simulink model "simulaciontorque"  (R2020b)
settings: Solver=VariableStepAuto  StartTime=0.0  StopTime=1.3  RelTol=1e-3
values from neighbouring files (symbols this model uses):
  beq = bm+(blnom/(r^2))    (= 1.5e-05)    [valores.m]
  Cts = 0.818    [Valores_de_Parametros.m]    (also in valores.m)
  Jeq = (Jm+Jl/r^2)    (= 5.65099476805e-06)    [Valores_de_Parametros.m]    (also in valores.m)
  lambda_m = 0.01546    [Valores_de_Parametros.m]    (also in valores.m)
  Ld = 6.6    [Valores_de_Parametros.m]    (also in valores.m = 0.0066)
  Lls = 0.8    [Valores_de_Parametros.m]    (also in valores.m = 0.0008)
  Lq = 5.8    [Valores_de_Parametros.m]    (also in valores.m = 0.0058)
  Pp = 3    [Valores_de_Parametros.m]    (also in valores.m)
  r = 314.3008    [Valores_de_Parametros.m]    (also in valores.m)
  R0 = Lls*pi    (= 4)    [valores.m]
  Rd = Ld*pi    (= 33)    [valores.m]
  Rq = Lq*pi    (= 29)    [valores.m]
  Rs = 1.02    [Valores_de_Parametros.m]    (also in valores.m)
  Rts_amb = 146.7    [Valores_de_Parametros.m]    (also in valores.m)
undefined symbols (not defined in the file or in its folder): sigbuilder_block
settings Model: Creator=Matias  LastModifiedBy=Matias

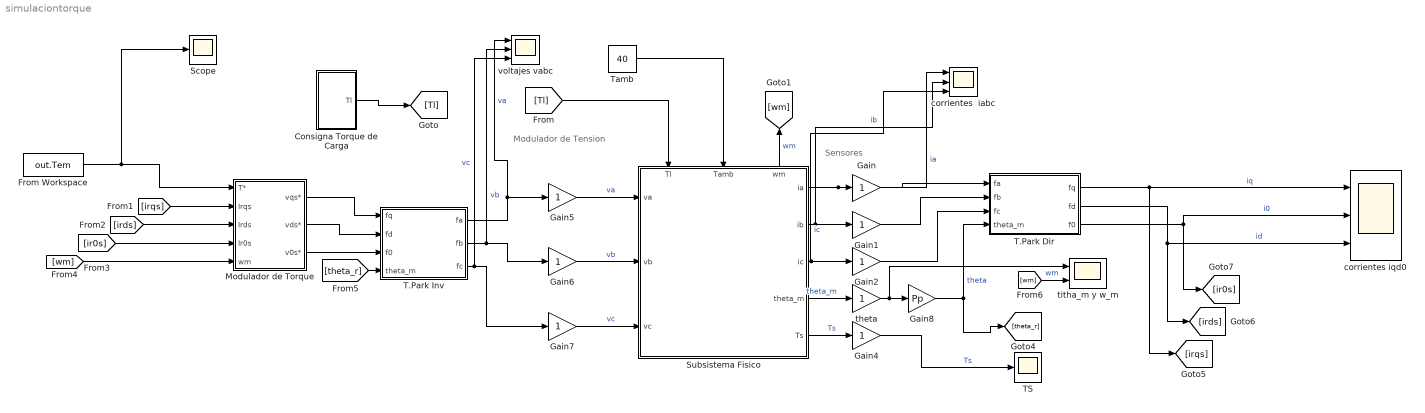
== system simulaciontorque ==
  note: Modulador de Tension
  note: Sensores
  Consigna Torque de Carga : Subsystem
  From Workspace : FromWorkspace  VariableName=out.Tem
  Gain{,1..2,4..7} (7 alike) : Gain
  Gain8 : Gain  Gain=Pp
  Modulador de Torque : Subsystem
  Scope : Scope
  Subsistema Fisico : Subsystem
      settings: PortSchema="{\"entries\":[{\"content\":{\"sides\":[{\"content\":{\"connectorIds\":[\"In1\",\"In2\",\"In3\"]},\"type\":\"ConnectorPlacement.EquallySpacedRectSide\",\"uuid\":\"428e53fe-c6d6-4999-95eb-db171c1d7752\"},{\"content\":{\"connectorIds\":[\"Out1\",\"Out2\",\"Out3\",\"Out4\",\"Out5\"],\"side\":\"RIGHT\"},\"type\":\"ConnectorPlacement.EquallySpacedRectSide\",\"uuid\":\"d3984cce-d898-4b9d-ab92-7967eebad5db\"},{\"content\":{\"connectorIds\":[\"In4\",\"In5\",\"Out6\"],\"side\":\"TOP\"},\"type\":\"ConnectorPlacement.EquallySpacedRectSide\",\"uuid\":\"4e08f4f3-ce82-4568-8c70-e26e1ed2ccd9\"},{\"content\":{\"connectorIds\":[],\"side\":\"BOTTOM\"},\"type\":\"ConnectorPlacement.EquallySpacedRectSide\",\"uuid\":\"f5359b7b-31c8-439d-9b4b-495d60398ac6\"},{\"content\":{\"connectorIds\":[],\"side\":\"HIDDEN\"},\"type\":\"ConnectorPlacement.EquallySpacedRectSide\",\"uuid\":\"fe5ef39c-0012-48bd-8627-0cf1abf153f6\"}]},\"type\":\"ConnectorPlacement.EquallySpacedConnector\",\"uuid\":\"3b2746a1-6d8c-49ea-8ba7-7e2e359e7a22\"}],\"packageUris\":[\"http://schema.mathworks.com/mf0/Connector/R2020b\"],\"version\":\"1.0\"}"
  T.Park Dir : MATLAB Function  TreatAsAtomicUnit=on
  T.Park Inv : MATLAB Function  TreatAsAtomicUnit=on
  TS : Scope
  Tamb : Constant  Value=40
  corrientes  iabc : Scope  NumInputPorts=3
  corrientes iqd0 : Scope  NumInputPorts=3
  theta : Gain
  titha_m y w_m : Scope  NumInputPorts=2
  voltajes vabc : Scope  NumInputPorts=3
  wires:
  Tamb/1 -> Subsistema Fisico/5(Tamb)
  [theta_r] -> T.Park Inv/4(theta_m)
  Modulador de Torque/1(vqs*) -> T.Park Inv/1(fq)
  [irds] -> Modulador de Torque/3(Irds)
  [ir0s] -> Modulador de Torque/4(Ir0s)
  Gain/1 -> T.Park Dir/1(fa)
  Modulador de Torque/2(vds*) -> T.Park Inv/2(fd)
  T.Park Inv/1(fa) -> voltajes vabc/1, Gain5/1  "va"
  T.Park Inv/2(fb) -> voltajes vabc/2, Gain6/1  "vb"
  [Tl] -> Subsistema Fisico/4(Tl)
  Gain4/1 -> TS/1  "Ts"
  theta/1 -> titha_m y w_m/1, Gain8/1
  T.Park Dir/2(fd) -> [irds], corrientes iqd0/3  "id"
  T.Park Dir/1(fq) -> [irqs], corrientes iqd0/1  "iq"
  Subsistema Fisico/1(ia) -> corrientes  iabc/1, Gain/1  "ia"
  Subsistema Fisico/2(ib) -> corrientes  iabc/2, Gain1/1  "ib"
  Gain5/1 -> Subsistema Fisico/1(va)  "va"
  Gain7/1 -> Subsistema Fisico/3(vc)  "vc"
  Subsistema Fisico/6(wm) -> [wm]  "wm"
  Gain6/1 -> Subsistema Fisico/2(vb)  "vb"
  T.Park Dir/3(f0) -> [ir0s], corrientes iqd0/2  "i0"
  T.Park Inv/3(fc) -> voltajes vabc/3, Gain7/1  "vc"
  Gain8/1 -> T.Park Dir/4(theta_m), [theta_r]  "theta"
  [wm] -> titha_m y w_m/2  "wm"
  Gain2/1 -> T.Park Dir/3(fc)
  Subsistema Fisico/3(ic) -> corrientes  iabc/3, Gain2/1  "ic"
  Subsistema Fisico/4(theta_m) -> theta/1  "theta_m"
  Subsistema Fisico/5(Ts) -> Gain4/1  "Ts"
  Modulador de Torque/3(v0s*) -> T.Park Inv/3(f0)
  [wm] -> Modulador de Torque/5(wm)
  Gain1/1 -> T.Park Dir/2(fb)
  [irqs] -> Modulador de Torque/2(Irqs)
  From Workspace/1 -> Scope/1, Modulador de Torque/1(T*)
  Consigna Torque de Carga/1(Tl) -> [Tl]

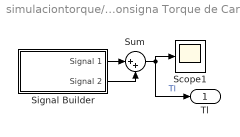
== system simulaciontorque/Consigna Torque de Carga ==
  Scope1 : Scope
  Signal Builder : Subsystem  Tag=STV Subsys  LoadFcn=sigbuilder_block('load');  StartFcn=sigbuilder_block('start');  StopFcn=sigbuilder_block('stop');  ClipboardFcn=sigbuilder_block('clipboard');  mask(Sigbuilder block){tuvar=[0:10]}
      mask help: Simulink:masks:SigbuilderBlock_MD
      mask init:
      | if ~strcmp(get_param(bdroot(gcbh),'SimulationStatus'),'stopped') tuvar = sigbuilder_block('maskInit'); end
      settings: CopyFcn=sigbuilder_block('copy');  DeleteFcn=sigbuilder_block('delete');  ModelCloseFcn=sigbuilder_block('modelClose');  PreSaveFcn=sigbuilder_block('preSave');  PauseFcn=sigbuilder_block('pause');  ContinueFcn=sigbuilder_block('continue');  NameChangeFcn=sigbuilder_block('namechange');  OpenFcn=sigbuilder_block('open',[388.2 64.2 550.8 400.2 ]);  CloseFcn=sigbuilder_block('close');
      mask Display: plot(0, 0, 100, 100,[2, 2, 32, 32, 2], [68, 8, 8, 68, 68],[32, 2], [38, 38], [32, 19, 2],[53, 60, 44], [32, 17, 17, 2],[16, 16, 31, 31]);txt = getActiveGroup(gcbh);text(2, 100, txt,'verticalAlignment', 'top');
  Sum : Sum  Inputs=|++
  Tl : Outport
  wires:
  Signal Builder/2(Signal 2) -> Sum/2
  Sum/1 -> Tl/1, Scope1/1  "Tl"
  Signal Builder/1(Signal 1) -> Sum/1

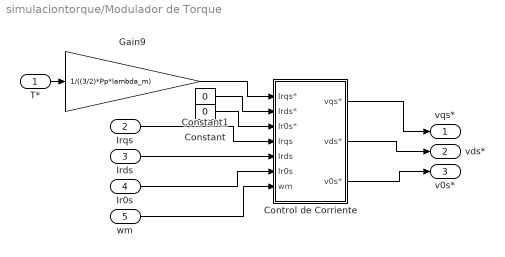
== system simulaciontorque/Modulador de Torque ==
  T* : Inport
  Irqs : Inport  Port=2
  Irds : Inport  Port=3
  Ir0s : Inport  Port=4
  wm : Inport  Port=5
  Constant : Constant  Value=0
  Constant1 : Constant  Value=0
  Control de Corriente : Subsystem
  Gain9 : Gain  Gain=1/((3/2)*Pp*lambda_m)
  vqs* : Outport
  vds* : Outport  Port=2
  v0s* : Outport  Port=3
  wires:
  Control de Corriente/2(vds*) -> vds*/1
  Irds/1 -> Control de Corriente/5(Irds)
  Gain9/1 -> Control de Corriente/1(Irqs*)
  Ir0s/1 -> Control de Corriente/6(Ir0s)
  Constant/1 -> Control de Corriente/3(Ir0s*)
  Control de Corriente/3(v0s*) -> v0s*/1
  Constant1/1 -> Control de Corriente/2(Irds*)
  Control de Corriente/1(vqs*) -> vqs*/1
  wm/1 -> Control de Corriente/7(wm)
  Irqs/1 -> Control de Corriente/4(Irqs)
  T*/1 -> Gain9/1

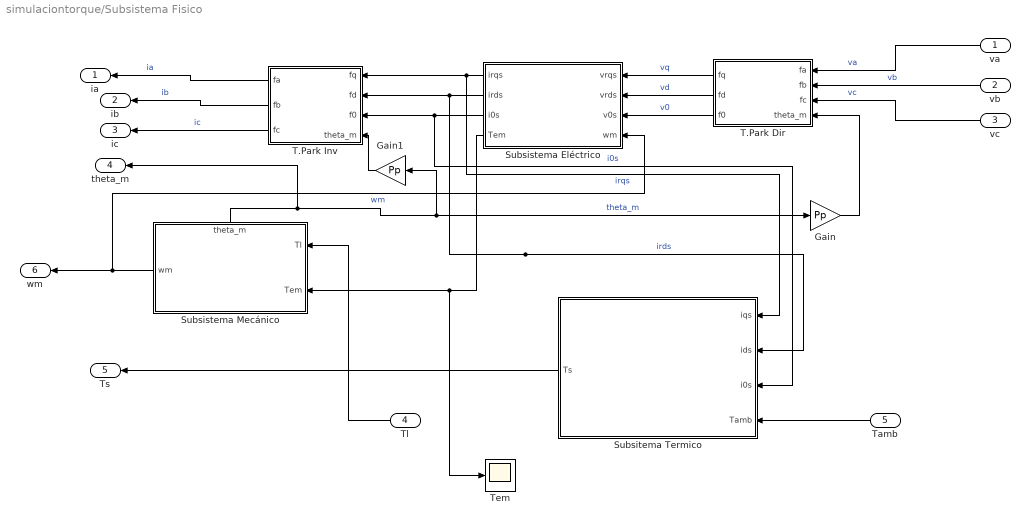
== system simulaciontorque/Subsistema Fisico ==
  va : Inport
  vb : Inport  Port=2
  vc : Inport  Port=3
  Tl : Inport  Port=4
  Tamb : Inport  Port=5
  Gain : Gain  Gain=Pp
  Gain1 : Gain  Gain=Pp
  Subsistema Eléctrico : Subsystem
  Subsistema Mecánico : Subsystem
      settings: PortSchema="{\"entries\":[{\"content\":{\"sides\":[{\"content\":{\"connectorIds\":[\"In1\",\"In2\"]},\"type\":\"ConnectorPlacement.EquallySpacedRectSide\",\"uuid\":\"ee0e19e9-1195-452b-ab3d-8be3dd040414\"},{\"content\":{\"connectorIds\":[\"Out1\"],\"side\":\"RIGHT\"},\"type\":\"ConnectorPlacement.EquallySpacedRectSide\",\"uuid\":\"524e54e6-4967-4b42-ae12-58774e9397a0\"},{\"content\":{\"connectorIds\":[\"Out2\"],\"side\":\"TOP\"},\"type\":\"ConnectorPlacement.EquallySpacedRectSide\",\"uuid\":\"fab71378-68cb-4446-b02c-df48705d1789\"},{\"content\":{\"connectorIds\":[],\"side\":\"HIDDEN\"},\"type\":\"ConnectorPlacement.EquallySpacedRectSide\",\"uuid\":\"eea92cb8-3517-43ef-96fe-10b46f054d59\"}]},\"type\":\"ConnectorPlacement.EquallySpacedConnector\",\"uuid\":\"156d3ac5-e5c7-4248-8590-4f82c7370a76\"}],\"packageUris\":[\"http://schema.mathworks.com/mf0/Connector/R2020b\"],\"version\":\"1.0\"}"
  Subsitema Termico : Subsystem
  T.Park Dir : MATLAB Function  TreatAsAtomicUnit=on
  T.Park Inv : MATLAB Function  TreatAsAtomicUnit=on
  Tem : Scope
  ia : Outport
  ib : Outport  Port=2
  ic : Outport  Port=3
  theta_m : Outport  Port=4
  Ts : Outport  Port=5
  wm : Outport  Port=6
  wires:
  Subsitema Termico/1(Ts) -> Ts/1
  Tl/1 -> Subsistema Mecánico/1(Tl)
  T.Park Inv/3(fc) -> ic/1  "ic"
  vb/1 -> T.Park Dir/2(fb)  "vb"
  Tamb/1 -> Subsitema Termico/4(Tamb)
  T.Park Inv/1(fa) -> ia/1  "ia"
  Subsistema Mecánico/1(wm) -> Subsistema Eléctrico/4(wm), wm/1  "wm"
  T.Park Dir/1(fq) -> Subsistema Eléctrico/1(vrqs)  "vq"
  Subsistema Eléctrico/3(i0s) -> Subsitema Termico/3(i0s), T.Park Inv/3(f0)  "i0s"
  Subsistema Eléctrico/1(irqs) -> Subsitema Termico/1(iqs), T.Park Inv/1(fq)  "irqs"
  Subsistema Eléctrico/2(irds) -> Subsitema Termico/2(ids), T.Park Inv/2(fd)  "irds"
  T.Park Dir/3(f0) -> Subsistema Eléctrico/3(v0s)  "v0"
  T.Park Dir/2(fd) -> Subsistema Eléctrico/2(vrds)  "vd"
  vc/1 -> T.Park Dir/3(fc)  "vc"
  T.Park Inv/2(fb) -> ib/1  "ib"
  Subsistema Mecánico/2(theta_m) -> theta_m/1, Gain1/1, Gain/1  "theta_m"
  va/1 -> T.Park Dir/1(fa)  "va"
  Subsistema Eléctrico/4(Tem) -> Tem/1, Subsistema Mecánico/2(Tem)
  Gain/1 -> T.Park Dir/4(theta_m)
  Gain1/1 -> T.Park Inv/4(theta_m)

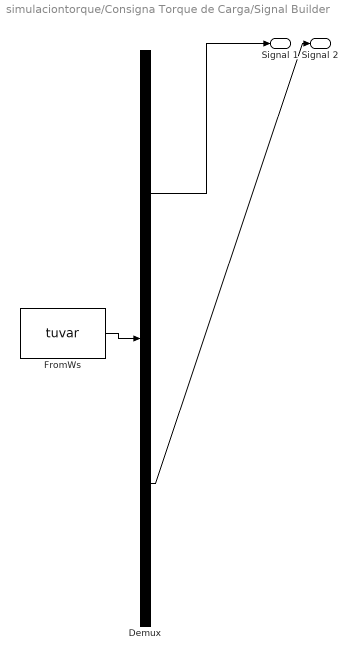
== system simulaciontorque/Consigna Torque de Carga/Signal Builder ==
  Demux : Demux  Tag=STV Demux  Outputs=2
      settings: DisplayOption=none
  FromWs : FromWorkspace  Tag=STV FromWs  VariableName=tuvar
      SigBuilderData=|
      | common.afterFinalStr = 'Extrapolate'
      | common.sampleTime = 0
      | dataSet.timeRange = [0 10]
      | dataSet.name = 'Group 1'
      | sbobj.Groups.Name = 'Group 1'
      | sbobj.Groups.Signals(1).Name = 'Signal 1'
      | sbobj.Groups.Signals(1).XData = [0 0.3 0.3 0.5 0.5 0.9 10]
      | sbobj.Groups.Signals(1).YData = [0 0 6.28 6.28 0 0 0]
      | sbobj.Groups.Signals(2).Name = 'Signal 2'
      | sbobj.Groups.Signals(2).XData = [0 0.5 0.5 0.9 0.9 10]
      | sbobj.Groups.Signals(2).YData = [0 0 -6.28 -6.28 0 0]
  Signal 1 : Outport  Tag=STV Outport
  Signal 2 : Outport  Tag=STV Outport  Port=2
  wires:
  Demux/1 -> Signal 1/1
  FromWs/1 -> Demux/1
  Demux/2 -> Signal 2/1

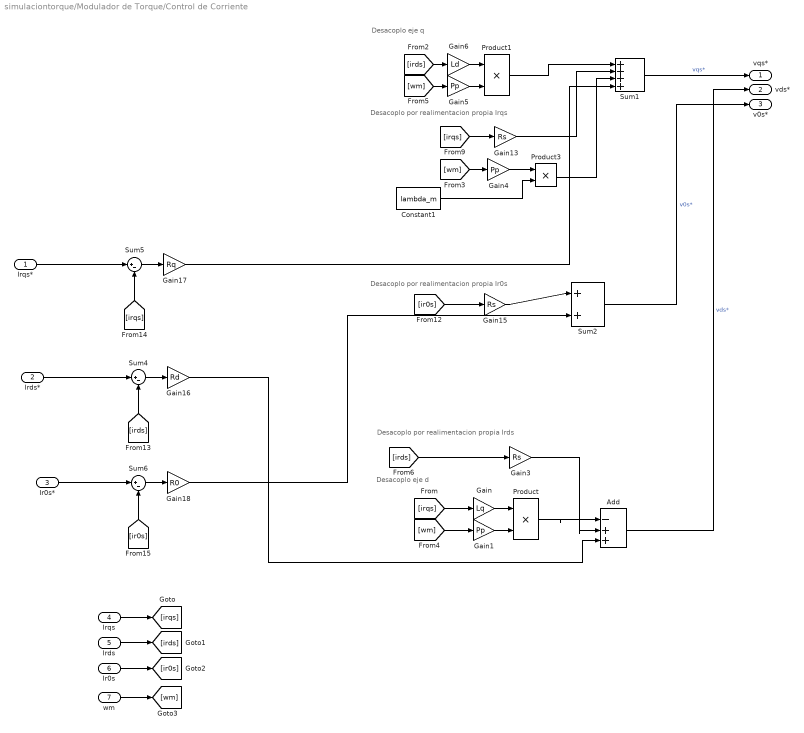
== system simulaciontorque/Modulador de Torque/Control de Corriente ==
  note: Desacoplo por realimentacion propia Ir0s
  note: Desacoplo por realimentacion propia Irqs
  note: Desacoplo por realimentacion propia Irds
  note: Desacoplo eje d
  note: Desacoplo eje q
  Irqs* : Inport
  Irds* : Inport  Port=2
  Ir0s* : Inport  Port=3
  Irqs : Inport  Port=4
  Irds : Inport  Port=5
  Ir0s : Inport  Port=6
  wm : Inport  Port=7
  Add : Sum  Inputs=|-++
  Constant1 : Constant  Value=lambda_m
  Gain : Gain  Gain=Lq
  Gain1 : Gain  Gain=Pp
  Gain13 : Gain  Gain=Rs
  Gain15 : Gain  Gain=Rs
  Gain16 : Gain  Gain=Rd
  Gain17 : Gain  Gain=Rq
  Gain18 : Gain  Gain=R0
  Gain3 : Gain  Gain=Rs
  Gain4 : Gain  Gain=Pp
  Gain5 : Gain  Gain=Pp
  Gain6 : Gain  Gain=Ld
  Product : Product
  Product1 : Product
  Product3 : Product
  Sum1 : Sum  Inputs=|++++
  Sum2 : Sum  Inputs=|++
  Sum4 : Sum  Inputs=|+-
  Sum5 : Sum  Inputs=|+-
  Sum6 : Sum  Inputs=|+-
  vqs* : Outport
  vds* : Outport  Port=2
  v0s* : Outport  Port=3
  wires:
  [ir0s] -> Sum6/2
  Sum2/1 -> v0s*/1  "v0s*"
  Irqs*/1 -> Sum5/1
  Ir0s*/1 -> Sum6/1
  Gain3/1 -> Add/2
  [irqs] -> Gain13/1
  [irds] -> Sum4/2
  [ir0s] -> Gain15/1
  Sum5/1 -> Gain17/1
  [irqs] -> Sum5/2
  [irds] -> Gain3/1
  Gain13/1 -> Sum1/2
  Sum6/1 -> Gain18/1
  Irds*/1 -> Sum4/1
  Gain15/1 -> Sum2/1
  Gain18/1 -> Sum2/2
  Gain17/1 -> Sum1/4
  Product1/1 -> Sum1/1
  Product/1 -> Add/1
  Gain5/1 -> Product1/2
  Gain/1 -> Product/1
  Gain4/1 -> Product3/1
  Sum4/1 -> Gain16/1
  Constant1/1 -> Product3/2
  Product3/1 -> Sum1/3
  Add/1 -> vds*/1  "vds*"
  Sum1/1 -> vqs*/1  "vqs*"
  Irqs/1 -> [irqs]
  Irds/1 -> [irds]
  Ir0s/1 -> [ir0s]
  [irqs] -> Gain/1
  Gain1/1 -> Product/2
  [wm] -> Gain1/1
  wm/1 -> [wm]
  [wm] -> Gain4/1
  [wm] -> Gain5/1
  [irds] -> Gain6/1
  Gain6/1 -> Product1/1
  Gain16/1 -> Add/3

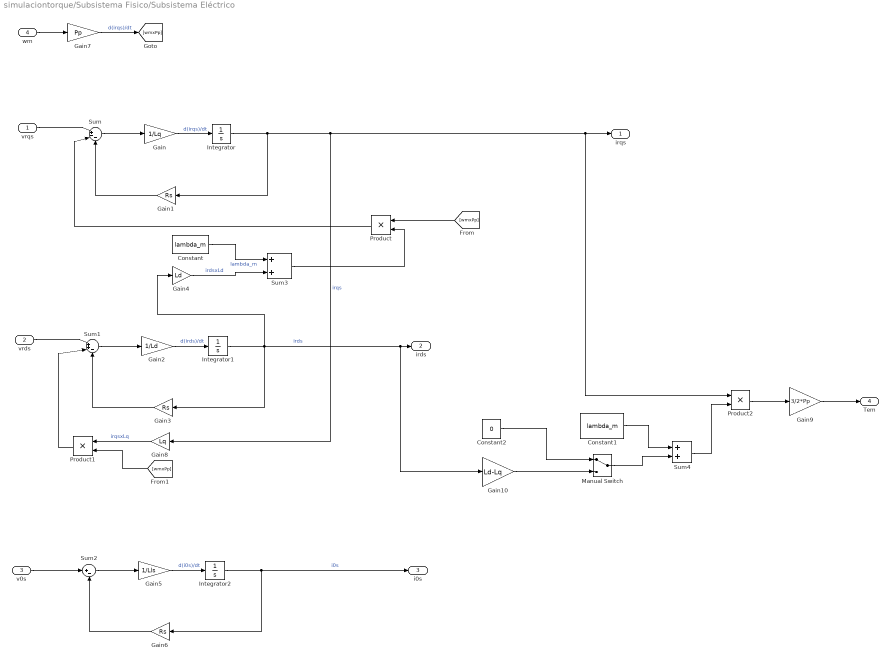
== system simulaciontorque/Subsistema Fisico/Subsistema Eléctrico ==
  vrqs : Inport
  vrds : Inport  Port=2
  v0s : Inport  Port=3
  wm : Inport  Port=4
  Constant : Constant  Value=lambda_m
  Constant1 : Constant  Value=lambda_m
  Constant2 : Constant  Value=0
  Gain : Gain  Gain=1/Lq
  Gain1 : Gain  Gain=Rs
  Gain10 : Gain  Gain=Ld-Lq
  Gain2 : Gain  Gain=1/Ld
  Gain3 : Gain  Gain=Rs
  Gain4 : Gain  Gain=Ld
  Gain5 : Gain  Gain=1/Lls
  Gain6 : Gain  Gain=Rs
  Gain7 : Gain  Gain=Pp
  Gain8 : Gain  Gain=Lq
  Gain9 : Gain  Gain=3/2*Pp
  Integrator : Integrator
  Integrator1 : Integrator
  Integrator2 : Integrator
  Manual Switch : ManualSwitch
  Product : Product
  Product1 : Product
  Product2 : Product
  Sum : Sum  Inputs=|+--
  Sum1 : Sum  Inputs=|++-
  Sum2 : Sum  Inputs=|+-
  Sum3 : Sum
  Sum4 : Sum
  irqs : Outport
  irds : Outport  Port=2
  i0s : Outport  Port=3
  Tem : Outport  Port=4
  wires:
  Integrator1/1 -> Gain4/1, Gain3/1, Gain10/1, irds/1  "irds"
  Gain2/1 -> Integrator1/1  "d(irds)/dt"
  Gain3/1 -> Sum1/3
  vrqs/1 -> Sum/1
  vrds/1 -> Sum1/1
  v0s/1 -> Sum2/1
  Gain5/1 -> Integrator2/1  "d(i0s)/dt"
  Integrator2/1 -> Gain6/1, i0s/1  "i0s"
  Gain1/1 -> Sum/3
  Integrator/1 -> Gain1/1, Gain8/1, Product2/1, irqs/1  "irqs"
  Gain/1 -> Integrator/1  "d(irqs)/dt"
  Gain6/1 -> Sum2/2
  Gain4/1 -> Sum3/2  "irdsxLd"
  Constant/1 -> Sum3/1  "lambda_m"
  wm/1 -> Gain7/1
  Gain7/1 -> [wmxPp]  "d(irqs)/dt"
  [wmxPp] -> Product/1
  Product/1 -> Sum/2
  Sum3/1 -> Product/2
  Gain8/1 -> Product1/1  "irqsxLq"
  [wmxPp] -> Product1/2
  Product1/1 -> Sum1/2
  Constant1/1 -> Sum4/1
  Sum4/1 -> Product2/2
  Product2/1 -> Gain9/1
  Gain9/1 -> Tem/1
  Sum/1 -> Gain/1
  Sum1/1 -> Gain2/1
  Sum2/1 -> Gain5/1
  Gain10/1 -> Manual Switch/2
  Constant2/1 -> Manual Switch/1
  Manual Switch/1 -> Sum4/2

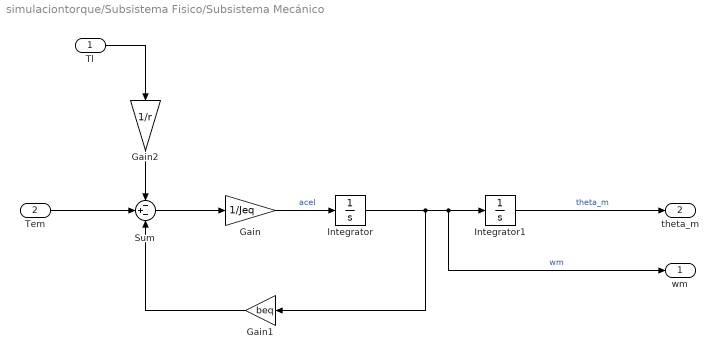
== system simulaciontorque/Subsistema Fisico/Subsistema Mecánico ==
  Tl : Inport
  Tem : Inport  Port=2
  Gain : Gain  Gain=1/Jeq
  Gain1 : Gain  Gain=beq
  Gain2 : Gain  Gain=1/r
  Integrator : Integrator
  Integrator1 : Integrator
  Sum : Sum  Inputs=-+-
  wm : Outport
  theta_m : Outport  Port=2
  wires:
  Sum/1 -> Gain/1
  Tl/1 -> Gain2/1
  Gain1/1 -> Sum/3
  Integrator/1 -> Gain1/1, wm/1, Integrator1/1  "wm"
  Gain2/1 -> Sum/1
  Gain/1 -> Integrator/1  "acel"
  Integrator1/1 -> theta_m/1  "theta_m"
  Tem/1 -> Sum/2

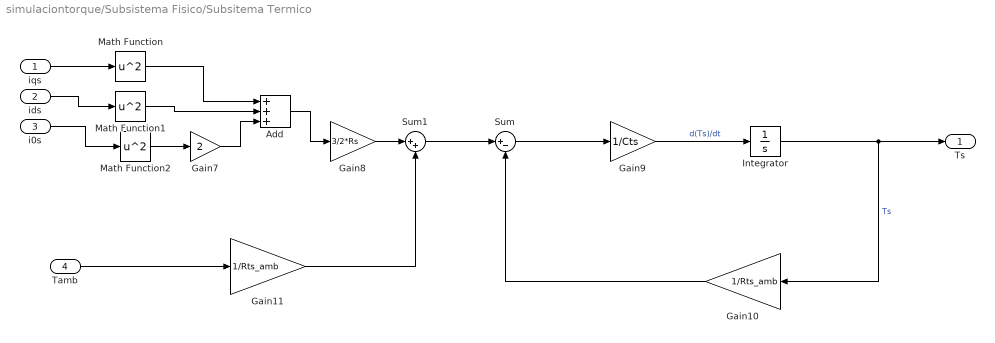
== system simulaciontorque/Subsistema Fisico/Subsitema Termico ==
  iqs : Inport
  ids : Inport  Port=2
  i0s : Inport  Port=3
  Tamb : Inport  Port=4
  Add : Sum  Inputs=+++
  Gain10 : Gain  Gain=1/Rts_amb
  Gain11 : Gain  Gain=1/Rts_amb
  Gain7 : Gain  Gain=2
  Gain8 : Gain  Gain=3/2*Rs
  Gain9 : Gain  Gain=1/Cts
  Integrator : Integrator  InitialCondition=40
  Math Function : Math  Operator=square  SaturateOnIntegerOverflow=on
  Math Function1 : Math  Operator=square  SaturateOnIntegerOverflow=on
  Math Function2 : Math  Operator=square  SaturateOnIntegerOverflow=on
  Sum : Sum  Inputs=|+-
  Sum1 : Sum  Inputs=|++
  Ts : Outport
  wires:
  Gain11/1 -> Sum1/2
  Gain8/1 -> Sum1/1
  Add/1 -> Gain8/1
  Gain9/1 -> Integrator/1  "d(Ts)/dt"
  Gain10/1 -> Sum/2
  Integrator/1 -> Gain10/1, Ts/1  "Ts"
  i0s/1 -> Math Function2/1
  Math Function/1 -> Add/1
  ids/1 -> Math Function1/1
  Sum1/1 -> Sum/1
  Gain7/1 -> Add/3
  Sum/1 -> Gain9/1
  Tamb/1 -> Gain11/1
  Math Function2/1 -> Gain7/1
  iqs/1 -> Math Function/1
  Math Function1/1 -> Add/2

== matlab function simulaciontorque/Subsistema Fisico/T.Park Dir ==
  data: fa input; fq output; fb input; fc input; theta_m input; fd output; f0 output
function [fq,fd,f0] = fcn(fa,fb,fc,theta_m)
fq=2/3*(cos(theta_m)*fa+cos(theta_m-(2*pi/(3)))*fb+cos(theta_m+(2*pi/(3)))*fc);
fd=2/3*(sin(theta_m)*fa+sin(theta_m-(2*pi/(3)))*fb+sin(theta_m+(2*pi/(3)))*fc);
f0=2/3*((1/2)*fa+(1/2)*fb+(1/2)*fc);

== matlab function simulaciontorque/Subsistema Fisico/T.Park Inv ==
  data: fq input; fa output; fd input; f0 input; theta_m input; fb output; fc output
function [fa,fb,fc] = fcn(fq,fd,f0,theta_m)
fa=fq*cos(theta_m)+fd*sin(theta_m)+f0;
fb=fq*cos(theta_m-(2*pi/(3)))+fd*sin(theta_m-(2*pi/(3)))+f0;
fc=fq*cos(theta_m+(2*pi/(3)))+fd*sin(theta_m+(2*pi/(3)))+f0;

== matlab function simulaciontorque/T.Park Dir ==
  data: fa input; fq output; fb input; fc input; theta_m input; fd output; f0 output
function [fq,fd,f0] = fcn(fa,fb,fc,theta_m)
fq=2/3*(cos(theta_m)*fa+cos(theta_m-(2*pi/(3)))*fb+cos(theta_m+(2*pi/(3)))*fc);
fd=2/3*(sin(theta_m)*fa+sin(theta_m-(2*pi/(3)))*fb+sin(theta_m+(2*pi/(3)))*fc);
f0=2/3*((1/2)*fa+(1/2)*fb+(1/2)*fc);

== matlab function simulaciontorque/T.Park Inv ==
  data: fq input; fa output; fd input; f0 input; theta_m input; fb output; fc output
function [fa,fb,fc] = fcn(fq,fd,f0,theta_m)
fa=fq*cos(theta_m)+fd*sin(theta_m)+f0;
fb=fq*cos(theta_m-(2*pi/(3)))+fd*sin(theta_m-(2*pi/(3)))+f0;
fc=fq*cos(theta_m+(2*pi/(3)))+fd*sin(theta_m+(2*pi/(3)))+f0;
